simulink model "GVCU_HIL"  (R2026a)
settings: Solver=ode3  StartTime=0  StopTime=2474  FixedStep=0.0002
model workspace (MAT data in the model file):
  CANoelibParameters.rawValue = 'off'
  CANoelibParameters.dataType = 'inherited'
  CANoelibParameters.checkTypeMismatch = 'Ignore'
  CANoelibParameters.sysvarStorageFile = 'canoelib.vsysvar'
  CANoelibParameters.fbRawValue = 'Physical value'
values from neighbouring files (symbols this model uses):
  acc_pedal_data = pedal_data.accelerator_pedal_position_t0    [Vehicle_Simulink_init.m]
  acc_pedal_time = pedal_data.t0    [Vehicle_Simulink_init.m]
  brk_pedal_data = brake_pedal_data.shared_brakes_drvrBrkPedlPerc_t0    [Vehicle_Simulink_init.m]
  brk_pedal_time = brake_pedal_data.t0    [Vehicle_Simulink_init.m]
  cycle_len = zeros(1, num_cycles)    [Vehicle_Simulink_init.m]
  cycle_speed_matrix = zeros(max_cycle_len, num_cycles)    [Vehicle_Simulink_init.m]
  cycle_time_matrix = zeros(max_cycle_len, num_cycles)    [Vehicle_Simulink_init.m]
  veh_speed_data = speed_data.shared_dynamicsVso_vehVelLgt_t0    [Vehicle_Simulink_init.m]
  veh_speed_time = speed_data.t0    [Vehicle_Simulink_init.m]
undefined symbols (not defined in the file or in its folder): Active, AuxActive, bat, environment, FL_prs_voltage, FR_prs_voltage, pos, RL_prs_voltage, RR_prs_voltage, tir, veh, VGetRawValueFlag, Voltage, VT2816_1_Ch1, VT2816_1_Ch2, VT2816_1_Ch3, VT2816_1_Ch4, VT2816_3_Ch13, VT2816_3_Ch14, VT7101_1_Out2, VT7820_2_Channel1, VT7820_2_Channel2, VT7820_2_Channel3, VT7820_2_Channel4, VTS
libraries: canoelib x144, autolibsharedcoupling x21, autolibcoupling x9, autolibshared x5, simulink_extras x4, simulink x4, slpidlib x3, autolibshareddiff x3, autolibutils x1, autolibdatasheetbattery x1, autolibmappedmotor x1, sl_discontinuities x1
(part 1 of 9)
settings Model: targetArch=x64  analysisModel=0  XcpMessageLength=-1  hasCAPLCallBlock=0  Creator=aakash.kavadimatti  LastModifiedBy=test.user1
settings DebuggingCC: InheritedTsInSrcMsg=none
settings RTWCC: SystemTargetFile=cn.tlc  TemplateMakefile=cn_msdll.tmf  Description=Vector CANoe Real-Time Target DLL (Visual C/C++ Project Makefile)
settings STFCustomTargetCC: SystemTargetFile=cn.tlc  MultiwordLength=2048.0  MatFileLogging=on  OutputDir=C:\work_local_TimBein\GVCU_HIL_repo\GVCU_HIL_Simulink_model\current_build  ExportCAPLFcn=off  ConnectOpenPorts=off  GenerateModelDescription=on  CheckCANoeBlockConfiguration=off  PerformSimStepAtStart=off  visualVersion=17.0  xcpEnableTimeStamp=0  PerformanceSysVars=off  canoeMatlabIFVersion=9.5.3  matlabVersionGreaterR2018b=1  debugBuildTlc=off  MIP_CONFIG_XCP_TIMESTAMPS_DISABLE=off  MIP_CONFIG_DISABLE_SYSVAR_WRITE_OPTIMIZATION=off  TargetArchitecture=Standard 64 Bit Real-Time DLL  SuppressCreateSVs=off  x64AnalysisModels=on  build64NodeLayerTlc=off  buildNodeLayerTlc=off  buildErtTlc=off  LegacyGuiDialogMappingPerformed=on  sampleTimesTlc=[0.001,0,0]  EnableParameterizationInReferencedModels=on  taskOverrunStrategyTlc=0.0  maxQueuedTasksTlc=0.0  EnableSignalAnalysis=on  EnableParameterization=on  MIP_CONFIG_IGNORE_NAN_UPDATES=off  EnableExcludeFromCANoeParameterization=off  MIP_CONFIG_SYSVAR_UPDATE_INTERVAL=-1.0  GenerateVModule=on  MIP_CONFIG_IS_APPLICATION_MODEL=off
settings GRTTargetCC: RTWCAPISignals=on  RTWCAPIParams=on  ParMdlRefBuildCompliant=off  CompOptLevelCompliant=off  ConcurrentExecutionCompliant=off  CombineOutputUpdateFcns=off  CPPClassGenCompliant=off  GRTInterface=on
settings SimscapeCC: SimscapeNominalValues="[{\"value\":\"1\",\"unit\":\"A\"},{\"value\":\"1\",\"unit\":\"bar\"},{\"value\":\"1\",\"unit\":\"cm^2\"},{\"value\":\"1\",\"unit\":\"cm^3/s\"},{\"value\":\"1\",\"unit\":\"kJ/kg\"},{\"value\":\"1\",\"unit\":\"kW\"},{\"value\":\"1\",\"unit\":\"l\"},{\"value\":\"1\",\"unit\":\"N\"},{\"value\":\"1\",\"unit\":\"N*m\"},{\"value\":\"1\",\"unit\":\"V\"}]"  SimscapeLogType=none  SimscapeLogDataHistory=5000.0

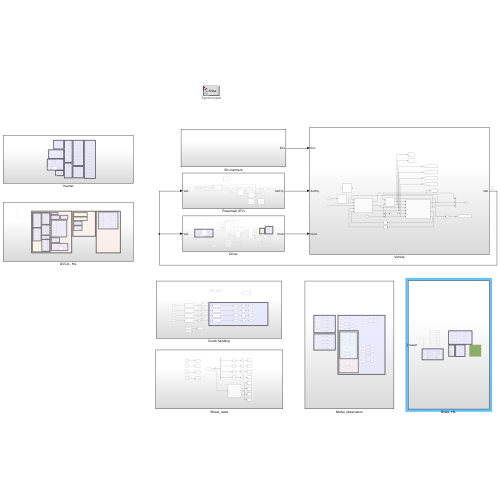
[thumbnail: Simulink's stored preview of the top-level diagram]
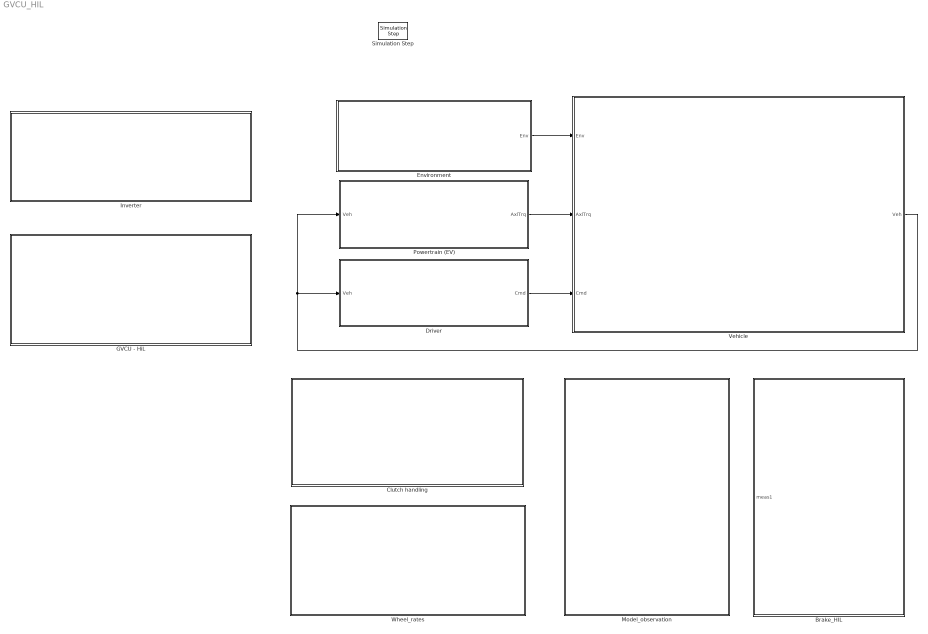
== system GVCU_HIL ==
  Brake_HIL : Subsystem
  Clutch handling : Subsystem
  Driver : Subsystem
  Environment : Subsystem
  GVCU - HiL : Subsystem
  Inverter : Subsystem
  Model_observation : Subsystem
  Powertrain (EV) : Subsystem
  Simulation Step : canoelib/CANoe I//O/Simulation Step  mode=Synchronized
      settings: AttributesFormatString=%<mode>  SourceProductName=Vector CANoe
  Vehicle : Subsystem
  Wheel_rates : Subsystem
  wires:
  Environment/1(Env) -> Vehicle/1(Env)
  Powertrain (EV)/1(AxlTrq) -> Vehicle/2(AxlTrq)
  Vehicle/1(Veh) -> Powertrain (EV)/1(Veh), Driver/1(Veh)
  Driver/1(Cmd) -> Vehicle/3(Cmd)

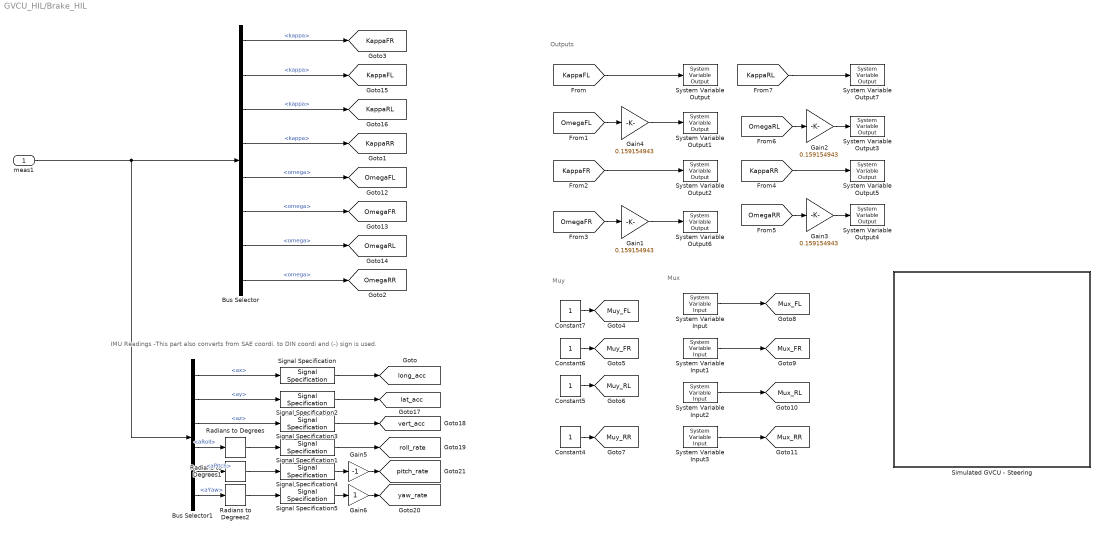
== system GVCU_HIL/Brake_HIL ==
  note: Outputs
  note: Muy
  note: Mux
  note: IMU Readings -This part also converts from SAE coordi. to DIN coordi and (-) sign is used.
  meas1 : Inport
  Bus Selector : BusSelector  OutputSignals=vehicle.front.right.tire.kappa,vehicle.front.left.tire.kappa,vehicle.rear.right.tire.kappa,vehicle.rear.left.tire.kappa,vehicle.front.left.tire.omega,vehicle.front.right.tire.omega,vehicle.rear.left.tire.omega,vehicle.rear.right.tire.omega
  Bus Selector1 : BusSelector  OutputSignals=vehicle.veh.local.ax,vehicle.veh.local.ay,vehicle.veh.local.az,vehicle.veh.global.aRoll,vehicle.veh.global.aPitch,vehicle.veh.global.aYaw
  Constant{4..7} (4 alike) : Constant
  Gain{1..4} (4 alike) : Gain  Gain=0.159154943
  Gain5 : Gain  Gain=-1
  Gain6 : Gain
  Radians to Degrees : simulink_extras/Transformations/Radians to Degrees
  Radians to Degrees1 : simulink_extras/Transformations/Radians to Degrees
  Radians to Degrees2 : simulink_extras/Transformations/Radians to Degrees
  Signal Specification : SignalSpecification  OutMin=[-65.532]  OutMax=[65.532]  Unit=m/s^2
  Signal Specification1 : SignalSpecification  OutMin=[-163.83]  OutMax=[163.83]  Unit=deg/s
  Signal Specification2 : SignalSpecification  OutMin=[-65.532]  OutMax=[65.532]  Unit=m/s^2
  Signal Specification3 : SignalSpecification  OutMin=[-65.532]  OutMax=[65.532]  Unit=m/s^2
  Signal Specification4 : SignalSpecification  OutMin=[-163.83]  OutMax=[163.83]  Unit=deg/s
  Signal Specification5 : SignalSpecification  OutMin=[-163.83]  OutMax=[163.83]  Unit=deg/s
  "Simulated GVCU - Steering " : Subsystem
  System Variable Input : canoelib/CANoe I//O/System Variable Input  nsName=ABS_TEST  sysVarName=Mux_FL  arrayIndex=-1  editSampleTime=0  rawValue=Default  dataType=Default  dataTypeDB=double  hasEncoding=off  dataTypeCANoe=Get from CANoe
      settings: AttributesFormatString=%<nsName>::%<sysVarName>  SourceProductName=Vector CANoe
  System Variable Input1 : canoelib/CANoe I//O/System Variable Input  nsName=ABS_TEST  sysVarName=Mux_FR  arrayIndex=-1  editSampleTime=0  rawValue=Default  dataType=Default  dataTypeDB=double  hasEncoding=off  dataTypeCANoe=Get from CANoe
      settings: AttributesFormatString=%<nsName>::%<sysVarName>  SourceProductName=Vector CANoe
  System Variable Input2 : canoelib/CANoe I//O/System Variable Input  nsName=ABS_TEST  sysVarName=Mux_RL  arrayIndex=-1  editSampleTime=0  rawValue=Default  dataType=Default  dataTypeDB=double  hasEncoding=off  dataTypeCANoe=Get from CANoe
      settings: AttributesFormatString=%<nsName>::%<sysVarName>  SourceProductName=Vector CANoe
  System Variable Input3 : canoelib/CANoe I//O/System Variable Input  nsName=ABS_TEST  sysVarName=Mux_RR  arrayIndex=-1  editSampleTime=0  rawValue=Default  dataType=Default  dataTypeDB=double  hasEncoding=off  dataTypeCANoe=Get from CANoe
      settings: AttributesFormatString=%<nsName>::%<sysVarName>  SourceProductName=Vector CANoe
  System Variable Output : canoelib/CANoe I//O/System Variable Output  nsName=ABS_TEST  sysVarName=kappa_FL  arrayIndex=-1  rawValue=Default  dataType=Default  dataTypeDB=double  hasEncoding=off  dataTypeCANoe=Get from CANoe
      settings: AttributesFormatString=%<nsName>::%<sysVarName>  SourceProductName=Vector CANoe
  System Variable Output1 : canoelib/CANoe I//O/System Variable Output  nsName=VTS::VT7820_2_Channel4  sysVarName=RotationFreq  arrayIndex=-1  rawValue=Default  dataType=Default  dataTypeDB=double  hasEncoding=off  dataTypeCANoe=Get from CANoe
      settings: AttributesFormatString=%<nsName>::%<sysVarName>  SourceProductName=Vector CANoe
  System Variable Output2 : canoelib/CANoe I//O/System Variable Output  nsName=ABS_TEST  sysVarName=Kappa_fr  arrayIndex=-1  rawValue=Default  dataType=Default  dataTypeDB=double  hasEncoding=off  dataTypeCANoe=Get from CANoe
      settings: AttributesFormatString=%<nsName>::%<sysVarName>  SourceProductName=Vector CANoe
  System Variable Output3 : canoelib/CANoe I//O/System Variable Output  nsName=VTS::VT7820_2_Channel1  sysVarName=RotationFreq  arrayIndex=-1  rawValue=Default  dataType=Default  dataTypeDB=double  hasEncoding=off  dataTypeCANoe=Get from CANoe
      settings: AttributesFormatString=%<nsName>::%<sysVarName>  SourceProductName=Vector CANoe
  System Variable Output4 : canoelib/CANoe I//O/System Variable Output  nsName=VTS::VT7820_2_Channel2  sysVarName=RotationFreq  arrayIndex=-1  rawValue=Default  dataType=Default  dataTypeDB=double  hasEncoding=off  dataTypeCANoe=Get from CANoe
      settings: AttributesFormatString=%<nsName>::%<sysVarName>  SourceProductName=Vector CANoe
  System Variable Output5 : canoelib/CANoe I//O/System Variable Output  nsName=ABS_TEST  sysVarName=Kappa_RR  arrayIndex=-1  rawValue=Default  dataType=Default  dataTypeDB=double  hasEncoding=off  dataTypeCANoe=Get from CANoe
      settings: AttributesFormatString=%<nsName>::%<sysVarName>  SourceProductName=Vector CANoe
  System Variable Output6 : canoelib/CANoe I//O/System Variable Output  nsName=VTS::VT7820_2_Channel3  sysVarName=RotationFreq  arrayIndex=-1  rawValue=Default  dataType=Default  dataTypeDB=double  hasEncoding=off  dataTypeCANoe=Get from CANoe
      settings: AttributesFormatString=%<nsName>::%<sysVarName>  SourceProductName=Vector CANoe
  System Variable Output7 : canoelib/CANoe I//O/System Variable Output  nsName=ABS_TEST  sysVarName=kappa_RL  arrayIndex=-1  rawValue=Default  dataType=Default  dataTypeDB=double  hasEncoding=off  dataTypeCANoe=Get from CANoe
      settings: AttributesFormatString=%<nsName>::%<sysVarName>  SourceProductName=Vector CANoe
  tag scope: KappaFL=global, KappaFR=global, KappaRL=global, KappaRR=global, Mux_FL=global, Mux_FR=global, Mux_RL=global, Mux_RR=global, Muy_FL=global, Muy_FR=global, Muy_RL=global, Muy_RR=global, OmegaFL=global, OmegaFR=global, OmegaRL=global, OmegaRR=global, lat_acc=global, long_acc=global, pitch_rate=global, roll_rate=global, vert_acc=global, yaw_rate=global
  wires:
  Gain2/1 -> System Variable Output3/1
  Constant5/1 -> [Muy_RL]
  [KappaRL] -> System Variable Output7/1
  System Variable Input3/1 -> [Mux_RR]
  [OmegaFL] -> Gain4/1
  System Variable Input/1 -> [Mux_FL]
  [OmegaRL] -> Gain2/1
  Constant4/1 -> [Muy_RR]
  [KappaRR] -> System Variable Output5/1
  [OmegaRR] -> Gain3/1
  [KappaFL] -> System Variable Output/1
  Constant7/1 -> [Muy_FL]
  Gain1/1 -> System Variable Output6/1
  [KappaFR] -> System Variable Output2/1
  Constant6/1 -> [Muy_FR]
  Gain3/1 -> System Variable Output4/1
  System Variable Input1/1 -> [Mux_FR]
  Gain4/1 -> System Variable Output1/1
  [OmegaFR] -> Gain1/1
  System Variable Input2/1 -> [Mux_RL]
  Bus Selector/5 -> [OmegaFL]  "<omega>"
  Bus Selector/1 -> [KappaFR]  "<kappa>"
  Bus Selector/8 -> [OmegaRR]  "<omega>"
  Bus Selector/2 -> [KappaFL]  "<kappa>"
  Bus Selector/3 -> [KappaRL]  "<kappa>"
  Bus Selector/4 -> [KappaRR]  "<kappa>"
  Bus Selector/7 -> [OmegaRL]  "<omega>"
  Bus Selector/6 -> [OmegaFR]  "<omega>"
  Signal Specification1/1 -> [roll_rate]
  Gain6/1 -> [yaw_rate]
  Radians to Degrees1/1 -> Signal Specification4/1
  Bus Selector1/6 -> Radians to Degrees2/1  "<aYaw>"
  Bus Selector1/3 -> Signal Specification3/1  "<az>"
  Bus Selector1/5 -> Radians to Degrees1/1  "<aPitch>"
  Bus Selector1/1 -> Signal Specification/1  "<ax>"
  Radians to Degrees/1 -> Signal Specification1/1
  Signal Specification3/1 -> [vert_acc]
  Bus Selector1/2 -> Signal Specification2/1  "<ay>"
  Gain5/1 -> [pitch_rate]
  meas1/1 -> Bus Selector1/1, Bus Selector/1
  Bus Selector1/4 -> Radians to Degrees/1  "<aRoll>"
  Signal Specification5/1 -> Gain6/1
  Radians to Degrees2/1 -> Signal Specification5/1
  Signal Specification2/1 -> [lat_acc]
  Signal Specification/1 -> [long_acc]
  Signal Specification4/1 -> Gain5/1

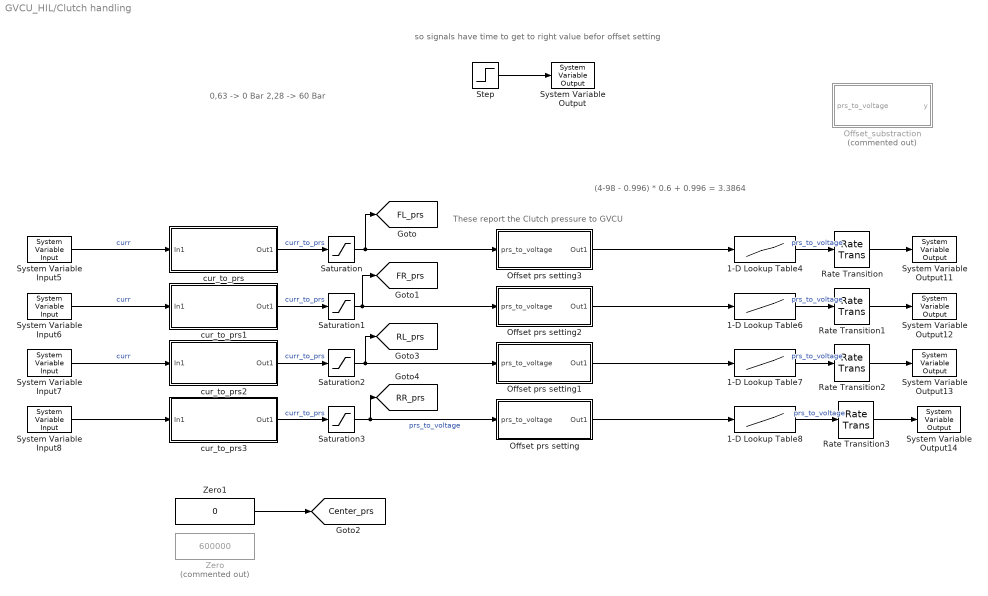
== system GVCU_HIL/Clutch handling ==
  note: so signals have time to get to right value befor offset setting
  note: (4-98 - 0.996) * 0.6 + 0.996 = 3.3864
  note: 0,63 -> 0 Bar
      | 2,28 -> 60 Bar
  note: These report the Clutch pressure to GVCU
  1-D Lookup Table{4,6..8} (4 alike) : Lookup_n-D  NumberOfTableDimensions=1  BreakpointsForDimension1=linspace(0,6000000,100)  Table=linspace(0.996,3.3864,100)  InternalRulePriority=Speed  RndMeth=Simplest
  Offset prs setting : Subsystem
  Offset prs setting1 : Subsystem
  Offset prs setting2 : Subsystem
  Offset prs setting3 : Subsystem
  Offset_substraction : Subsystem  Commented=on
  Rate Transition{,1..3} (4 alike) : RateTransition  OutPortSampleTime=0.005
  Saturation{,1..3} (4 alike) : Saturate  UpperLimit=10000000  LowerLimit=0
  Step : Step  Time=0.1  SampleTime=0
  System Variable Input5 : canoelib/CANoe I//O/System Variable Input  nsName=VTS::VT2816_1_Ch4  sysVarName=CurCurrent  arrayIndex=-1  editSampleTime=0  rawValue=Default  dataType=Default  dataTypeDB=double  hasEncoding=off  dataTypeCANoe=Get from CANoe
      settings: AttributesFormatString=%<nsName>::%<sysVarName>  SourceProductName=Vector CANoe
  System Variable Input6 : canoelib/CANoe I//O/System Variable Input  nsName=VTS::VT2816_1_Ch3  sysVarName=CurCurrent  arrayIndex=-1  editSampleTime=0  rawValue=Default  dataType=Default  dataTypeDB=double  hasEncoding=off  dataTypeCANoe=Get from CANoe
      settings: AttributesFormatString=%<nsName>::%<sysVarName>  SourceProductName=Vector CANoe
  System Variable Input7 : canoelib/CANoe I//O/System Variable Input  nsName=VTS::VT2816_1_Ch2  sysVarName=CurCurrent  arrayIndex=-1  editSampleTime=0  rawValue=Default  dataType=Default  dataTypeDB=double  hasEncoding=off  dataTypeCANoe=Get from CANoe
      settings: AttributesFormatString=%<nsName>::%<sysVarName>  SourceProductName=Vector CANoe
  System Variable Input8 : canoelib/CANoe I//O/System Variable Input  nsName=VTS::VT2816_1_Ch1  sysVarName=CurCurrent  arrayIndex=-1  editSampleTime=0  rawValue=Default  dataType=Default  dataTypeDB=double  hasEncoding=off  dataTypeCANoe=Get from CANoe
      settings: AttributesFormatString=%<nsName>::%<sysVarName>  SourceProductName=Vector CANoe
  System Variable Output : canoelib/CANoe I//O/System Variable Output  nsName=VTS::VT7101_1_Out2  sysVarName=Active  arrayIndex=-1  rawValue=Default  dataType=Default  dataTypeDB=int32  hasEncoding=off  dataTypeCANoe=Get from CANoe
      settings: AttributesFormatString=%<nsName>::%<sysVarName>  SourceProductName=Vector CANoe
  System Variable Output11 : canoelib/CANoe I//O/System Variable Output  nsName=VTS  sysVarName=FL_prs_voltage::Voltage  arrayIndex=-1  rawValue=Default  dataType=Default  dataTypeDB=double  hasEncoding=off  dataTypeCANoe=Get from CANoe
      settings: AttributesFormatString=%<nsName>::%<sysVarName>  SourceProductName=Vector CANoe
  System Variable Output12 : canoelib/CANoe I//O/System Variable Output  nsName=VTS  sysVarName=FR_prs_voltage::Voltage  arrayIndex=-1  rawValue=Default  dataType=Default  dataTypeDB=double  hasEncoding=off  dataTypeCANoe=Get from CANoe
      settings: AttributesFormatString=%<nsName>::%<sysVarName>  SourceProductName=Vector CANoe
  System Variable Output13 : canoelib/CANoe I//O/System Variable Output  nsName=VTS  sysVarName=RL_prs_voltage::Voltage  arrayIndex=-1  rawValue=Default  dataType=Default  dataTypeDB=double  hasEncoding=off  dataTypeCANoe=Get from CANoe
      settings: AttributesFormatString=%<nsName>::%<sysVarName>  SourceProductName=Vector CANoe
  System Variable Output14 : canoelib/CANoe I//O/System Variable Output  nsName=VTS  sysVarName=RR_prs_voltage::Voltage  arrayIndex=-1  rawValue=Default  dataType=Default  dataTypeDB=double  hasEncoding=off  dataTypeCANoe=Get from CANoe
      settings: AttributesFormatString=%<nsName>::%<sysVarName>  SourceProductName=Vector CANoe
  Zero : Constant  Commented=on  Value=600000  OutDataTypeStr=Inherit: Inherit via back propagation
  Zero1 : Constant  Value=0  OutDataTypeStr=Inherit: Inherit via back propagation
  cur_to_prs : Subsystem
  cur_to_prs1 : Subsystem
  cur_to_prs2 : Subsystem
  cur_to_prs3 : Subsystem
  tag scope: Center_prs=global, FL_prs=global, FR_prs=global, RL_prs=global, RR_prs=global
  wires:
  System Variable Input8/1 -> cur_to_prs3/1(In1)
  cur_to_prs1/1(Out1) -> Saturation1/1  "curr_to_prs"
  cur_to_prs2/1(Out1) -> Saturation2/1  "curr_to_prs"
  cur_to_prs/1(Out1) -> Saturation/1  "curr_to_prs"
  System Variable Input5/1 -> cur_to_prs/1(In1)  "curr"
  1-D Lookup Table7/1 -> Rate Transition2/1  "prs_to_voltage"
  Zero1/1 -> [Center_prs]
  cur_to_prs3/1(Out1) -> Saturation3/1  "curr_to_prs"
  Saturation3/1 -> [RR_prs], Offset prs setting/1(prs_to_voltage)  "prs_to_voltage"
  System Variable Input6/1 -> cur_to_prs1/1(In1)  "curr"
  System Variable Input7/1 -> cur_to_prs2/1(In1)  "curr"
  1-D Lookup Table4/1 -> Rate Transition/1  "prs_to_voltage"
  1-D Lookup Table6/1 -> Rate Transition1/1  "prs_to_voltage"
  Rate Transition/1 -> System Variable Output11/1
  Rate Transition1/1 -> System Variable Output12/1
  Rate Transition2/1 -> System Variable Output13/1
  Rate Transition3/1 -> System Variable Output14/1
  Saturation/1 -> Offset prs setting3/1(prs_to_voltage), [FL_prs]
  Saturation1/1 -> Offset prs setting2/1(prs_to_voltage), [FR_prs]
  Saturation2/1 -> Offset prs setting1/1(prs_to_voltage), [RL_prs]
  1-D Lookup Table8/1 -> Rate Transition3/1  "prs_to_voltage"
  Step/1 -> System Variable Output/1
  Offset prs setting3/1(Out1) -> 1-D Lookup Table4/1
  Offset prs setting2/1(Out1) -> 1-D Lookup Table6/1
  Offset prs setting1/1(Out1) -> 1-D Lookup Table7/1
  Offset prs setting/1(Out1) -> 1-D Lookup Table8/1

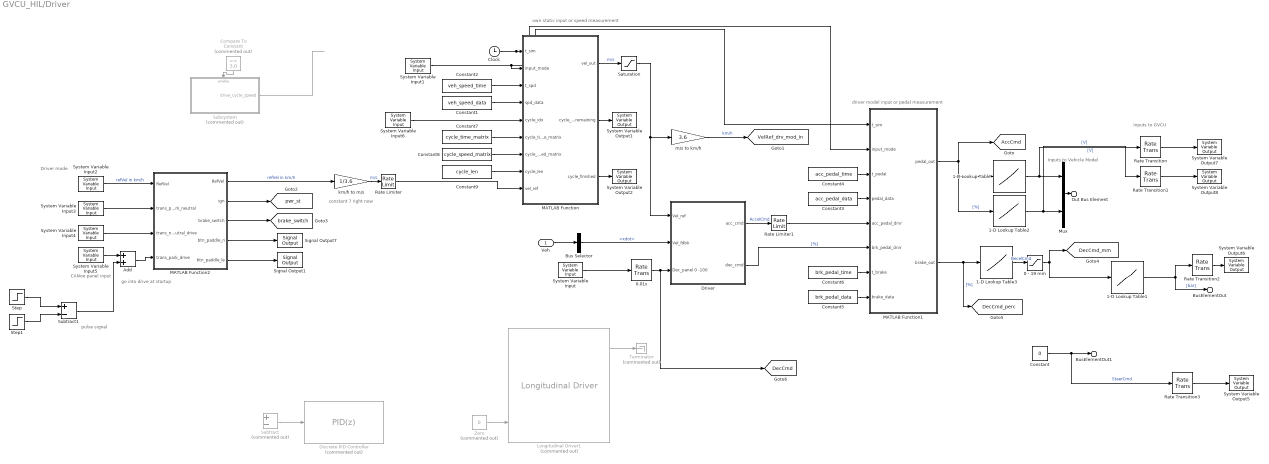
== system GVCU_HIL/Driver ==
  note: pulse signal
  note: go into drive at startup
  note: own static input or speed measurement
  note: CANoe panel input
  note: constant 7 right now
  note: Driver mode
  note: Inputs to GVCU
  note: Inputs to Vehicle Model
  note: driver model input or pedal measurement
  Veh : Inport
  0 - 19 mm : Saturate  UpperLimit=19  LowerLimit=0
  0.01s : RateTransition  OutPortSampleTime=0.01
  1-D Lookup Table : Lookup_n-D  NumberOfTableDimensions=1  BreakpointsForDimension1=linspace(0,100,100)  Table=linspace(0.4,2.0,100)  InternalRulePriority=Speed  RndMeth=Simplest
  1-D Lookup Table1 : Lookup_n-D  NumberOfTableDimensions=1  BreakpointsForDimension1="[0,  2,  4,  6,  8,  10, 12, 14,  16,  19 ]"  Table="[0,  7,  12, 16, 22, 32, 48, 72,  105, 180]"  InternalRulePriority=Speed  RndMeth=Simplest
  1-D Lookup Table2 : Lookup_n-D  NumberOfTableDimensions=1  BreakpointsForDimension1=linspace(0,100,100)  Table=linspace(0.8,4.0,100)  InternalRulePriority=Speed  RndMeth=Simplest
  1-D Lookup Table3 : Lookup_n-D  NumberOfTableDimensions=1  BreakpointsForDimension1=[0 22.9 45.3 45.8]  Table=[0 5.1 10.1 10.3]  InternalRulePriority=Speed  RndMeth=Simplest
  Add : Sum
  Bus Selector : BusSelector  OutputSignals=Body.BdyFrm.Cg.Vel.xdot
  Clock : Clock
  Compare To Constant : simulink/Logic and Bit Operations/Compare To Constant  Commented=on  relop===  const=3.0  OutDataTypeStr=boolean
  Constant : Constant  Value=0
  Constant1 : Constant  Value=veh_speed_data
  Constant2 : Constant  Value=veh_speed_time
  Constant3 : Constant  Value=acc_pedal_data
  Constant4 : Constant  Value=acc_pedal_time
  Constant5 : Constant  Value=brk_pedal_data
  Constant6 : Constant  Value=brk_pedal_time
  Constant7 : Constant  Value=cycle_time_matrix
  Constant8 : Constant  Value=cycle_speed_matrix
  Constant9 : Constant  Value=cycle_len
  Discrete PID Controller : slpidlib/PID Controller  Commented=on  Controller=PID  Form=Parallel  TimeDomain=Discrete-time  UseExternalTs=off  SampleTime=-1  IntegratorMethod=Forward Euler  FilterMethod=Forward Euler  ControllerParametersSource=internal  P=500  I=10  UseKiTs=off  D=0  UseExternalDerivativeSource=off  N=100  UseFilter=on  TunerSelectOption=Transfer Function Based (PID Tuner App)  InitialConditionSource=internal  InitialConditionForIntegrator=0  InitialConditionForFilter=0  DifferentiatorICPrevScaledInput=0  ExternalReset=none  TrackingMode=off  Kt=1  LimitOutput=off  SatLimitsSource=internal  UpperSaturationLimit=inf  LowerSaturationLimit=-inf  LinearizeAsGain=off  AntiWindupMode=none  Kb=1  LimitIntegrator=off  UpperIntegratorSaturationLimit=inf  LowerIntegratorSaturationLimit=-inf  POutMin=[]  POutMax=[]  IOutMin=[]  IOutMax=[]  DOutMin=[]  DOutMax=[]  NOutMin=[]  NOutMax=[]  SumOutMin=[]  SumOutMax=[]  SaturationOutMin=[]  SaturationOutMax=[]  PParamMin=[]  PParamMax=[]  IParamMin=[]  IParamMax=[]  DParamMin=[]  DParamMax=[]  NParamMin=[]  NParamMax=[]  KbParamMin=[]  KbParamMax=[]  KtParamMin=[]  KtParamMax=[]  KbOutMin=[]  KbOutMax=[]  KtOutMin=[]  KtOutMax=[]  IntegratorOutMin=[]  IntegratorOutMax=[]  FilterOutMin=[]  FilterOutMax=[]  SumI1OutMin=[]  SumI1OutMax=[]  SumI2OutMin=[]  SumI2OutMax=[]  SumI3OutMin=[]  SumI3OutMax=[]  SumI4OutMin=[]  SumI4OutMax=[]  SumDOutMin=[]  SumDOutMax=[]  DifferentiatorOutMin=[]  DifferentiatorOutMax=[]  FilterDiffOutCoefMin=[]  FilterDiffOutCoefMax=[]  ReciprocalOutMin=[]  ReciprocalOutMax=[]  SumDenOutMin=[]  SumDenOutMax=[]  SumNumOutMin=[]  SumNumOutMax=[]  DivideOutMin=[]  DivideOutMax=[]  UdiffTsProdOutMin=[]  UdiffTsProdOutMax=[]  NTsProdOutMin=[]  NTsProdOutMax=[]  UintegralTsProdOutMin=[]  UintegralTsProdOutMax=[]  UngainTsProdOutMin=[]  UngainTsProdOutMax=[]  ClampingZeroOutDataTypeStr=Inherit: Inherit via back propagation  ClampingZeroOutMin=[]  ClampingZeroOutMax=[]  FilterDenConstantOutDataTypeStr=Inherit: Inherit via back propagation  FilterDenConstantOutMin=[]  FilterDenConstantOutMax=[]  PCopyOutDataTypeStr=Inherit: Inherit via back propagation  PCopyOutMin=[]  PCopyOutMax=[]  NCopyOutDataTypeStr=Inherit: Inherit via back propagation  NCopyOutMin=[]  NCopyOutMax=[]  IntegratorContinuousStateAttributes=''  IntegratorStateMustResolveToSignalObject=off  IntegratorRTWStateStorageClass=Auto  FilterContinuousStateAttributes=''  FilterStateMustResolveToSignalObject=off  FilterRTWStateStorageClass=Auto  ParallelPVariant=InternalParameters  IdealPVariant=Disabled  IVariant=InternalParameters  DVariant=InternalParameters  IntegratorVariant=Discrete  SatVariant=Disabled  AWVariant=Passthrough  PCopyVariant=Disabled  TRVariant=Disabled  FdbkBlocksVariant=Forward  IdealPFdbkVariant=Disabled  SatFdbkVariant=Disabled  DerivativeFilterVariant=ForwardEulerFilter  NVariant=InternalParameters  NCopyVariant=Disabled  FilterICVariant=InternalICsFilter  IntegratorICVariant=InternalICs  ExternalResetVariant=Disabled  TRSumVariant=Passthrough  SumFdbkVariant=Disabled  SumVariant=Sum_PID  TsampFilterVariant=InternalTs  TsampNgainVariant=Passthrough  TsampIntegralVariant=Disabled_SignalSpec  ExternalSaturationOutDataTypeStr=Inherit: Same as second input  DerivativeSourceVariant=ErrorSignal  PreIntVariant=InternalPreInt
      settings: LibrarySourceBlock=simulink/Discrete/Discrete PID Controller
  Driver : Subsystem
  Longitudinal Driver1 : autolibshared/Longitudinal Driver  Commented=on  extAccelOvr=off  extDecelOvr=off  extAccelHld=off  extDecelHld=off  extAccelZero=off  extDecelZero=off  cntrlType=PI  shftType=None  velUnits=m/s  gearOut=off  Kp=10  Ki=1  Kff=.2  Kg=.01  VehVelVec=[0 70]  KffVec=[.12 .4]  KpVec=[25 10]  KiVec=[0.5 0.2]  KgVec=[0 0]  m=1500  Kpt=3000  tau=.1  L=2  aR=200  bR=2.5  cR=veh.aero.CD  g=9.81  vnom=35  Kaw=1  tauerr=.03  tauPt=2  GearInit=0  tShift=.1  pdlVec=[0.1 0.4 0.5 0.9]  upShftTbl=[-1 12.9375 26.4375 39.9375 51.18749999999999 62.4375 72.84375 83.25;-1 16.3125 29.8125 43.3125 54.5624 65.8125 76.78125 87.75;-1 19.6875 33.1875 46.68749999999999 57.9375 69.1875 80.71875 92.25;-1 33 52.5 77.25 100.5 138.75 161.875 185]  dwnShftTbl=[1 9.5625 23.0625 36.5625 47.8125 59.0625 68.90625 78.75;1 12.9375 26.4375 39.9375 51.18749999999999 62.4375 72.84375 83.25;1 16.3125 29.8125 43.3125 54.562499 65.8125 76.78125 87.75;1 19.6875 33.1875 46.68749999999999 57.9375 69.1875 80.71875 92.25]  tClutch=.5  tRev=.5  tPark=120  aMode=1  UpGearVec="[0  1  2  3  4  5  6  7]"  DownGearVec="[1  2  3  4  5  6  7  8]"
  MATLAB Function : MATLAB Function  TreatAsAtomicUnit=on
  MATLAB Function1 : MATLAB Function  TreatAsAtomicUnit=on
  MATLAB Function2 : MATLAB Function  TreatAsAtomicUnit=on
  Mux : Mux  Inputs=2
  Rate Limiter : RateLimiter  RisingSlewLimit=20  FallingSlewLimit=-20  SampleTimeMode=inherited
  Rate Limiter1 : RateLimiter  RisingSlewLimit=50  FallingSlewLimit=-50  SampleTimeMode=inherited
  Rate Transition{,1..3} (4 alike) : RateTransition  OutPortSampleTime=0.01
  Saturation : Saturate  UpperLimit=1000  LowerLimit=0
  Signal Output1 : canoelib/CANoe I//O/Signal Output  dbName=main_bus  nodeName=HPDM2  msgName=steer_whl_repack  sigName=btn_paddle_le  rawValue=Default  dataType=Default  dataTypeDB=uint8  hasEncoding=off
      settings: AttributesFormatString=%<sigName>  SourceProductName=Vector CANoe
  Signal Output7 : canoelib/CANoe I//O/Signal Output  dbName=main_bus  nodeName=HPDM2  msgName=steer_whl_repack  sigName=btn_paddle_ri  rawValue=Default  dataType=Default  dataTypeDB=uint8  hasEncoding=off
      settings: AttributesFormatString=%<sigName>  SourceProductName=Vector CANoe
  Step : Step  Time=0.4
  Step1 : Step  Time=0.45
  Subsystem : Subsystem  Commented=on
  Subtract : Sum  Commented=on  Inputs=+-
  Subtract1 : Sum  Inputs=+-
  System Variable Input : canoelib/CANoe I//O/System Variable Input  nsName=Checker_Simulink  sysVarName=Panel_brake_pedal_perc  arrayIndex=-1  editSampleTime=0  rawValue=Default  dataType=Default  dataTypeDB=int32  hasEncoding=off  dataTypeCANoe=Get from CANoe
      settings: AttributesFormatString=%<nsName>::%<sysVarName>  SourceProductName=Vector CANoe
  System Variable Input1 : canoelib/CANoe I//O/System Variable Input  nsName=Checker_Simulink  sysVarName=input_mode  arrayIndex=-1  editSampleTime=0  rawValue=Default  dataType=Default  dataTypeDB=int32  hasEncoding=off  dataTypeCANoe=Get from CANoe
      settings: AttributesFormatString=%<nsName>::%<sysVarName>  SourceProductName=Vector CANoe
  System Variable Input2 : canoelib/CANoe I//O/System Variable Input  nsName=Checker_Simulink  sysVarName=RefVel  arrayIndex=-1  editSampleTime=0  rawValue=Default  dataType=Default  dataTypeDB=int32  hasEncoding=off  dataTypeCANoe=Get from CANoe
      settings: AttributesFormatString=%<nsName>::%<sysVarName>  SourceProductName=Vector CANoe
  System Variable Input3 : canoelib/CANoe I//O/System Variable Input  nsName=drive_mode_requests  sysVarName=trans_park_neutral  arrayIndex=-1  editSampleTime=0  rawValue=Default  dataType=Default  dataTypeDB=int32  hasEncoding=off  dataTypeCANoe=Get from CANoe
      settings: AttributesFormatString=%<nsName>::%<sysVarName>  SourceProductName=Vector CANoe
  System Variable Input4 : canoelib/CANoe I//O/System Variable Input  nsName=drive_mode_requests  sysVarName=trans_neutral_drive  arrayIndex=-1  editSampleTime=0  rawValue=Default  dataType=Default  dataTypeDB=int32  hasEncoding=off  dataTypeCANoe=Get from CANoe
      settings: AttributesFormatString=%<nsName>::%<sysVarName>  SourceProductName=Vector CANoe
  System Variable Input5 : canoelib/CANoe I//O/System Variable Input  nsName=drive_mode_requests  sysVarName=trans_park_drive  arrayIndex=-1  editSampleTime=0  rawValue=Default  dataType=Default  dataTypeDB=int32  hasEncoding=off  dataTypeCANoe=Get from CANoe
      settings: AttributesFormatString=%<nsName>::%<sysVarName>  SourceProductName=Vector CANoe
  System Variable Input6 : canoelib/CANoe I//O/System Variable Input  nsName=Checker_Simulink  sysVarName=drive_cycle_idx  arrayIndex=-1  editSampleTime=0  rawValue=Default  dataType=Default  dataTypeDB=int32  hasEncoding=off  dataTypeCANoe=Get from CANoe
      settings: AttributesFormatString=%<nsName>::%<sysVarName>  SourceProductName=Vector CANoe
  System Variable Output1 : canoelib/CANoe I//O/System Variable Output  nsName=Checker_Simulink  sysVarName=cycle_time_left  arrayIndex=-1  rawValue=Default  dataType=Default  dataTypeDB=int32  hasEncoding=off  dataTypeCANoe=Get from CANoe
      settings: AttributesFormatString=%<nsName>::%<sysVarName>  SourceProductName=Vector CANoe
  System Variable Output2 : canoelib/CANoe I//O/System Variable Output  nsName=Checker_Simulink  sysVarName=cycle_finished  arrayIndex=-1  rawValue=Default  dataType=Default  dataTypeDB=int32  hasEncoding=off  dataTypeCANoe=Get from CANoe
      settings: AttributesFormatString=%<nsName>::%<sysVarName>  SourceProductName=Vector CANoe
  System Variable Output5 : canoelib/CANoe I//O/System Variable Output  nsName=VehicleRefVel  sysVarName=SteerCmd  arrayIndex=-1  rawValue=Default  dataType=Default  dataTypeDB=int32  hasEncoding=off  dataTypeCANoe=Get from CANoe
      settings: AttributesFormatString=%<nsName>::%<sysVarName>  SourceProductName=Vector CANoe
  System Variable Output6 : canoelib/CANoe I//O/System Variable Output  nsName=VehicleRefVel  sysVarName=DecelCmd  arrayIndex=-1  rawValue=Default  dataType=Default  dataTypeDB=int32  hasEncoding=off  dataTypeCANoe=Get from CANoe
      settings: AttributesFormatString=%<nsName>::%<sysVarName>  SourceProductName=Vector CANoe
  System Variable Output7 : canoelib/CANoe I//O/System Variable Output  nsName=VTS  sysVarName=VT2816_3_Ch14::Voltage  arrayIndex=-1  rawValue=Default  dataType=Default  dataTypeDB=double  hasEncoding=off  dataTypeCANoe=Get from CANoe
      settings: AttributesFormatString=%<nsName>::%<sysVarName>  SourceProductName=Vector CANoe
  System Variable Output8 : canoelib/CANoe I//O/System Variable Output  nsName=VTS  sysVarName=VT2816_3_Ch13::Voltage  arrayIndex=-1  rawValue=Default  dataType=Default  dataTypeDB=double  hasEncoding=off  dataTypeCANoe=Get from CANoe
      settings: AttributesFormatString=%<nsName>::%<sysVarName>  SourceProductName=Vector CANoe
  Terminator : Terminator  Commented=on
  Zero : Constant  Commented=on  Value=0  OutDataTypeStr=Inherit: Inherit via back propagation
  km/h to m/s : Gain  Gain=1/3.6
  m/s to km/h : Gain  Gain=3.6
  Out Bus Element : Outport  Description=Throttle pedal position  VectorParamsAs1DForOutWhenUnconnected=off  PortName=Cmd  Element=AccelCmd
  BusElementOut : Outport  Description=Brake pedal position  PortName=Cmd  Element=DecelCmd
  BusElementOut1 : Outport  Description=Steering wheel angle  PortName=Cmd  Element=SteerCmd
  tag scope: AccCmd=global, DecCmd=global, DecCmd_mm=global, DecCmd_perc=global, VelRef_drv_mod_in=global, brake_switch=global, pwr_st=global
  wires:
  Zero/1 -> Longitudinal Driver1/3
  Veh/1 -> Bus Selector/1
  Bus Selector/1 -> Driver/2(Vel_fdbk)  "<xdot>"
  Constant/1 -> Rate Transition3/1, BusElementOut1/1  "SteerCmd"
  Longitudinal Driver1/1 -> Terminator/1
  1-D Lookup Table1/1 -> BusElementOut/1, Rate Transition2/1  "[bar]"
  1-D Lookup Table2/1 -> Rate Transition1/1, Mux/2  "[V]"
  Mux/1 -> Out Bus Element/1
  Rate Limiter/1 -> MATLAB Function/9(vel_ref)
  MATLAB Function2/1(RefVel) -> km/h to m/s/1  "refVel in km/h"
  System Variable Input3/1 -> MATLAB Function2/2(trans_park_neutral)
  MATLAB Function2/5(btn_paddle_le) -> Signal Output1/1
  MATLAB Function2/4(btn_paddle_ri) -> Signal Output7/1
  Add/1 -> MATLAB Function2/4(trans_park_drive)
  MATLAB Function2/2(ign) -> [pwr_st]
  System Variable Input4/1 -> MATLAB Function2/3(trans_neutral_drive)
  MATLAB Function2/3(brake_switch) -> [brake_switch]
  System Variable Input2/1 -> MATLAB Function2/1("RefVel ")  "refVel in km/h"
  1-D Lookup Table/1 -> Rate Transition/1, Mux/1  "[V]"
  Rate Transition/1 -> System Variable Output7/1
  Rate Transition1/1 -> System Variable Output8/1
  Rate Transition2/1 -> System Variable Output6/1
  Rate Transition3/1 -> System Variable Output5/1
  1-D Lookup Table3/1 -> 0 - 19 mm/1  "DecelCmd"
  km/h to m/s/1 -> Rate Limiter/1  "m/s"
  System Variable Input1/1 -> MATLAB Function1/2(input_mode), MATLAB Function/2(input_mode)
  MATLAB Function/1(vel_out) -> Saturation/1  "m/s"
  m/s to km/h/1 -> [VelRef_drv_mod_in]  "km/h"
  MATLAB Function1/1(pedal_out) -> 1-D Lookup Table2/1, 1-D Lookup Table/1, [AccCmd]  "[%]"
  Saturation/1 -> Driver/1(Vel_ref), m/s to km/h/1
  Clock/1 -> MATLAB Function1/1(t_sim), MATLAB Function/1(t_sim)
  Constant1/1 -> MATLAB Function/4(spd_data)
  Constant2/1 -> MATLAB Function/3(t_spd)
  Driver/1(acc_cmd) -> Rate Limiter1/1  "AccelCmd"
  Constant4/1 -> MATLAB Function1/3(t_pedal)
  Constant3/1 -> MATLAB Function1/4(pedal_data)
  MATLAB Function1/2(brake_out) -> [DecCmd_perc], 1-D Lookup Table3/1  "[%]"
  Constant5/1 -> MATLAB Function1/8(brake_data)
  Constant6/1 -> MATLAB Function1/7(t_brake)
  Subtract/1 -> Discrete PID Controller/1
  System Variable Input6/1 -> MATLAB Function/5(cycle_idx)
  System Variable Input/1 -> 0.01s/1
  0.01s/1 -> [DecCmd], Driver/3(Dec_panel 0 -100)
  Driver/2(dec_cmd) -> MATLAB Function1/6(brk_pedal_drvr)  "[%]"
  0 - 19 mm/1 -> [DecCmd_mm], 1-D Lookup Table1/1
  Rate Limiter1/1 -> MATLAB Function1/5(acc_pedal_drvr)
  System Variable Input5/1 -> Add/1
  Step/1 -> Subtract1/1
  Step1/1 -> Subtract1/2
  Subsystem/1(drive_cycle_speed) -> ?
  Compare To Constant/1 -> Subsystem/Enable
  Constant7/1 -> MATLAB Function/6(cycle_time_matrix)
  Constant8/1 -> MATLAB Function/7(cycle_speed_matrix)
  Constant9/1 -> MATLAB Function/8(cycle_len)
  MATLAB Function/2(cycle_time_remaining) -> System Variable Output1/1
  MATLAB Function/3(cycle_finished) -> System Variable Output2/1
  Subtract1/1 -> Add/2

== system GVCU_HIL/Environment ==
  Air : Subsystem
  Bus Creator : BusCreator  Inputs=4
  Friction : Subsystem
  Ground : Subsystem
  Wind : Subsystem
  Env : Outport
  tag scope: Env=global
  wires:
  Bus Creator/1 -> [Env], Env/1
  Ground/1(Ground) -> Bus Creator/4  "Ground"
  Wind/1(Wind) -> Bus Creator/1  "Wind"
  Air/1(Air) -> Bus Creator/2  "Air"
  Friction/1(Friction) -> Bus Creator/3  "Friction"
